simulink model "AEB4"  (R2024b)
settings: Solver=FixedStepAuto  StartTime=0.0  StopTime=10.0  RelTol=1e-3
undefined symbols (not defined in the file or in its folder): camera, gray
libraries: visionanalysis x1
settings Model: Creator=csamak  LastModifiedBy=tsamak
settings OptimizationCC: ZeroExternalMemoryAtStartup=off  ZeroInternalMemoryAtStartup=off  InitFltsAndDblsToZero=on
settings HardwareCC: ProdLongLongMode=on  TargetLongLongMode=on
settings SFSimCC: SimTargetLang=C++
settings RTWCC: TargetLang=C++  GenerateGPUCode=CUDA
settings GRTTargetCC: TargetLangStandard=C++11 (ISO)  CodeInterfacePackaging=C++ class

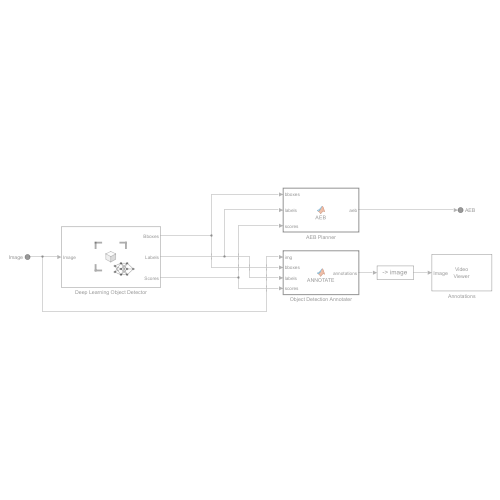
[thumbnail: Simulink's stored preview of the top-level diagram]
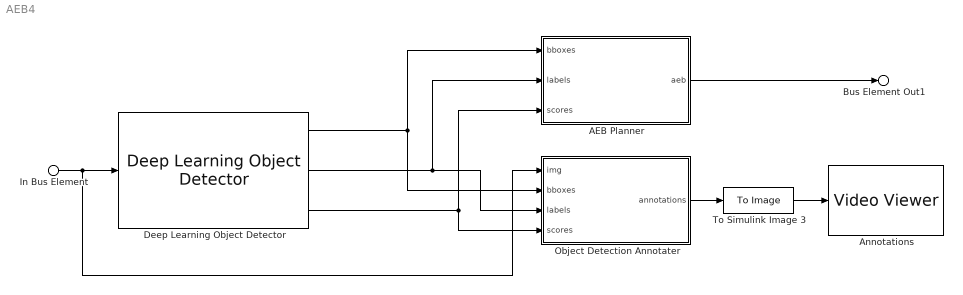
== system AEB4 ==
  In Bus Element : Inport  PortName=Image
  AEB Planner : MATLAB Function  TreatAsAtomicUnit=on
  Annotations : VideoViewer  colormapValue=gray(256)  FigPos=[1241.66666666667 442 408 253.333333333333]
  Deep Learning Object Detector : visionanalysis/Deep Learning Object Detector  Detector=Detector from MAT-file  DetectorFunction=vehicleDetectorYOLOv2  DetectorFilePath=C:\Users\tsamak\Downloads\MathWorks RZR AEB - System Composer\yolov3.mat  MaxDetections=7  Bboxes=on  Scores=on  UseROI=off  AutoResize=on  ROI=[1 1 camera.ImageSize(2) round(camera.ImageSize(1)*0.678)]  Threshold=0.4  NumStrongestRegions=2000  UseMinSize=off  MinSize=[1 1]  UseMaxSize=off  MaxSize=[50 50]  ForceInterpretedSim=off
  Object Detection Annotater : MATLAB Function  TreatAsAtomicUnit=on
  To Simulink Image 3 : ToImage
  Bus Element Out1 : Outport  PortName=AEB
  wires:
  Deep Learning Object Detector/1 -> Object Detection Annotater/2(bboxes), AEB Planner/1(bboxes)
  Deep Learning Object Detector/2 -> Object Detection Annotater/3(labels), AEB Planner/2(labels)
  To Simulink Image 3/1 -> Annotations/1
  Deep Learning Object Detector/3 -> AEB Planner/3(scores), Object Detection Annotater/4(scores)
  Object Detection Annotater/1(annotations) -> To Simulink Image 3/1
  In Bus Element/1 -> Object Detection Annotater/1(img), Deep Learning Object Detector/1
  AEB Planner/1(aeb) -> Bus Element Out1/1

== matlab function AEB4/AEB Planner ==
  data: bboxes input; aeb output; labels input; scores input
function aeb = AEB(bboxes, labels, scores)
    aeb = 0;
    valid_labels = [yolov3_labels.bird_label, yolov3_labels.cat_label, ...
                    yolov3_labels.dog_label, yolov3_labels.horse_label, ...
                    yolov3_labels.sheep_label, yolov3_labels.cow_label, ...
                    yolov3_labels.elephant_label, yolov3_labels.bear_label, ...
                    yolov3_labels.zebra_label, yolov3_labels.giraffe_label];
    for i=1:size(bboxes,1)
        if (any(valid_labels(:) == labels(i)))
            if (scores(i) >= 0.5)
                if (bboxes(i,3)*bboxes(i,4) >= 4000)
                    aeb = 1;
                else
                    aeb = 0;
                end
            else
                aeb = 0;
            end
        else
            aeb = 0;
        end
    end

== matlab function AEB4/Object Detection Annotater ==
  data: img input; annotations output; bboxes input; labels input; scores input
function annotations = ANNOTATE(img, bboxes, labels, scores)
    annotations = uint8(zeros(360,640,3));
    annotations = insertObjectAnnotation(img,"rectangle",bboxes,labels);
